simulink model "GPSRead"  (Simulink 6.6)
settings: Solver=FixedStepDiscrete  StartTime=0.0  StopTime=10.0  FixedStep=0.001  RelTol=1e-3
InitFcn:
  | initGPS
undefined symbols (not defined in the file or in its folder): gpsInit, gpsParse, gpsRead, gpsSeparate, u1, uartInit, y1
libraries: dsPICdrivers x13, simulink x1, xpclib x1
settings Model: Creator=ASL_Lab  LastModifiedBy=ASL_Lab  ProdHWDeviceType=16-bit Generic
settings OptimizationCC: InlineParams=on  OptimizeModelRefInitCode=on  LifeSpan=1
settings HardwareCC: ProdBitPerInt=16  ProdEndianess=LittleEndian  ProdWordSize=16  ProdHWDeviceType=16-bit Generic  TargetHWDeviceType=32-bit Generic
settings RTWCC: SystemTargetFile=dspic.tlc  TemplateMakefile=dspic_pic30_gcc.tmf  PostCodeGenCommand=dsPIC_Compile()  Description=Embedded Target for Microchip dsPIC (real-time)  GenerateReport=on  ProcessScript=dspic_make_rtw_hook  IncludeHyperlinkInReport=on  LaunchReport=on
settings RTWCC: CustomSource=|
  | clib\circBuffer.c
  | clib\gpsParse.c
  | clib\gpsSplit.c
  | clib\sbrk.c
  | clib\bufferedUART.c
settings CodeAppCC: IgnoreCustomStorageClasses=off
settings STFCustomTargetCC: TargetFcnLib=ansi_tfl_tmw.mat  GenFloatMathFcnCalls=ANSI_C  ModelReferenceCompliant=off  IncludeMdlTerminateFcn=off  CombineOutputUpdateFcns=on  SuppressErrorStatus=on  ERTCustomFileBanners=on  SupportContinuousTime=off  SupportNonInlinedSFcns=off  SystemTargetFile=dspic.tlc
settings ERTTargetCC: TargetFcnLib=ansi_tfl_tmw.mat  GenFloatMathFcnCalls=ANSI_C  ModelReferenceCompliant=off  IncludeMdlTerminateFcn=off  SuppressErrorStatus=on  ModelStepFunctionPrototypeControlCompliant=off  ExtModeMexFile=noextcomm  InlinedParameterPlacement=NonHierarchical  ERTSrcFileBannerTemplate=dsPIC_code_template.cgt  ERTHdrFileBannerTemplate=dsPIC_code_template.cgt  ERTDataSrcFileTemplate=dsPIC_code_template.cgt  ERTDataHdrFileTemplate=dsPIC_code_template.cgt  ERTCustomFileTemplate=dsPIC_main.tlc
settings CustomProperty: DataType=string  Value=C:\PROGRA~1\MATLAB\R2007a\rtw\bin\win32\gmake

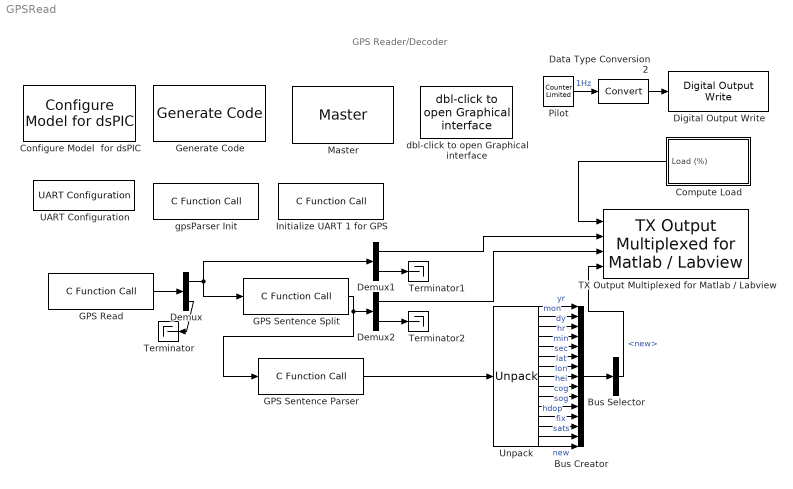
== system GPSRead ==
  note: GPS Reader/Decoder
  Bus Creator : BusCreator  Inputs=15
  Bus Selector : BusSelector  OutputSignals=new
  Compute Load : Subsystem  Orientation=left
  Configure Model  for dsPIC : dsPICdrivers/Simulink Configuration/Configure Model  for dsPIC
  Data Type Conversion2 : DataTypeConversion  OutDataTypeMode=boolean
  Demux : Demux  Outputs=[25 1]
  Demux1 : Demux  Outputs=[1 24]
  Demux2 : Demux  Outputs=[1 126]
  Digital Output Write : dsPICdrivers/Digital I//O/Digital Output Write  Tag=dsPIC_Digital_Output  Priority=5  PORT=G  Pin=[ 14]  Simultaneous=off  OrderingInOutPopup=None
  GPS Read : dsPICdrivers/OTHERS/C Function Call  Tag=dsPIC_dsPIC_CFunctionCall  fctName='gpsRead'  INPUT_SIZE=1  INPUT1=--  INPUT2=--  INPUT3=--  OUTPUT_SIZE=26  OUTPUT1=uint8  SampleTime=-1  InputType=[ ]  OutputType=[ 2 ]  FctDeclaration=extern void gpsRead(uint8_T* y1);  FctCall=gpsRead(*%y1);  OrderingInOutPopup=None
  GPS Sentence Parser : dsPICdrivers/OTHERS/C Function Call  Tag=dsPIC_dsPIC_CFunctionCall  fctName='gpsParse'  INPUT_SIZE=127  INPUT1=uint8  INPUT2=--  INPUT3=--  OUTPUT_SIZE=27  OUTPUT1=uint8  SampleTime=-1  InputType=[ 2 ]  OutputType=[ 2 ]  FctDeclaration=extern void gpsParse(uint8_T* u1,uint8_T* y1);  FctCall=gpsParse(*%u1, *%y1);  OrderingInOutPopup=None
  GPS Sentence Split : dsPICdrivers/OTHERS/C Function Call  Tag=dsPIC_dsPIC_CFunctionCall  fctName='gpsSeparate'  INPUT_SIZE=25  INPUT1=uint8  INPUT2=--  INPUT3=--  OUTPUT_SIZE=127  OUTPUT1=uint8  SampleTime=-1  InputType=[ 2 ]  OutputType=[ 2 ]  FctDeclaration=extern void gpsSeparate(uint8_T* u1,uint8_T* y1);  FctCall=gpsSeparate(*%u1, *%y1);  OrderingInOutPopup=None
  Generate Code : dsPICdrivers/Simulink Configuration/Generate Code
  Initialize UART 1 for GPS : dsPICdrivers/OTHERS/C Function Call  Tag=dsPIC_dsPIC_CFunctionCall  fctName='uartInit'  INPUT_SIZE=1  INPUT1=--  INPUT2=--  INPUT3=--  OUTPUT_SIZE=1  OUTPUT1=--  SampleTime=inf  InputType=[ ]  OutputType=[ ]  FctDeclaration=extern void uartInit();  FctCall=uartInit();  OrderingInOutPopup=None
  Master : dsPICdrivers/Master  Tag=dsPIC_MASTER  Priority=1  TimeStepType=Timer1  picType=33fJ256MC710  fcy=40000000  Quartz_33f=12e6  PLLActive_33f=on  fcyDesired_33f=40e6  tmr1="[1  39999  0]"  tmr1Info="Time Step : 0.001  ;   Error : 0%  PR1=39999"  tmr2345="[0  0  0  0  0  0  0  0]"  tmr2345cfg=[-1 -1 -1 -1 -1 -1 -1 -1]  IOautoConf=on  typePort="[ 0   0   0   0   0   0  10  10   0   0   0   0   0   0   0   0   0   0   0   0   0   0   0   0   0   0   0   0   0   0   0   0   0   0   0   0   0   0   0   0   0   0   0   0   0   0   0   0   0   0   0   0   0   0   0   0   0   0   0   0   0   0   0   0   0   0   0   0   0   0   0   0   0   0   0   0   0   0   0   0   0   0   0   0   4   5   0   0   0   0   0   0   0   0   0   0   0   0   0   0   0   0   0   0   0   0   0   0   0   0  10   0 ]"  TRIS="[ 65343  65535  65535  65535  65535  65535  49151 ]"  ADPCFG=12582912  MasterBusyPort=A7  MasterOverloadPort=A6  FOSC=Quartz (XT - HS)  TempProtection_33f=TEMP_ON  FPBOR=<empty>  PWRT=disable  MCLR=<empty>  PowerSave=off
  Pilot : simulink/Sources/Counter Limited  SystemSampleTime=-1  uplimit=1  tsamp=1.0
  TX Output Multiplexed for Matlab / Labview : dsPICdrivers/Serial PORT/TX Output Multiplexed for Matlab // Labview  Tag=dsPIC_TX_Multiplexed  Priority=5  UART=2  CleverSpreadingChk=on  CleverSpreading=1  CHANNEL="[0 1 2 3  ]"  CHANNELBLOCKED=[]  CHANNELBLOCKED_BITEWISE=0  Status=OK
  Terminator : Terminator
  Terminator1 : Terminator
  Terminator2 : Terminator
  UART Configuration : dsPICdrivers/Serial PORT/UART Configuration  Tag=dsPIC_config_UART  Priority=2  UART=2  proposed_BAUD=19200  ALT_TX_RX=off  InterruptTxWhen=When Transmit Buffer is empty  TXInterruptPri=6  TxBufferSize=64  TXEN=on  InterruptRxWhen=When Receive Buffer is full (contain 4 characters)  RXInterruptPri=5  RxBufferSize=64  BAUD=19200  UxBRG=129  Info="UxBRG = 129   ||  Real Baud : 19231   ||  % error : 0.16026  ||  max 1.9231 Bytes / Step"  RealBaud=0
  Unpack : xpclib/UDP/Unpack  dimensions={1,1,1,1,1,1,1,1,1,1,1,1,1,1,1}  datatypes={'uint8', 'uint8', 'uint8', 'uint8', 'uint8', 'uint8', 'single', 'single','single','uint16', 'uint16', 'uint16', 'uint8','uint8', 'uint8'}  byteAlign=1
  dbl-click to open Graphical interface : dsPICdrivers/Serial PORT/dbl-click to open Graphical interface  SystemSampleTime=-1  Nothing=0
  gpsParser Init : dsPICdrivers/OTHERS/C Function Call  Tag=dsPIC_dsPIC_CFunctionCall  fctName='gpsInit'  INPUT_SIZE=1  INPUT1=--  INPUT2=--  INPUT3=--  OUTPUT_SIZE=1  OUTPUT1=--  SampleTime=inf  InputType=[ ]  OutputType=[ ]  FctDeclaration=extern void gpsInit();  FctCall=gpsInit();  OrderingInOutPopup=None
  wires:
  Pilot/1 -> Data Type Conversion2/1  "1Hz"
  Data Type Conversion2/1 -> Digital Output Write/1
  Compute Load/1(Load (%)) -> TX Output Multiplexed for Matlab / Labview/1
  GPS Sentence Split/1 -> GPS Sentence Parser/1, Demux2/1
  GPS Sentence Parser/1 -> Unpack/1
  Unpack/1 -> Bus Creator/1  "yr"
  Unpack/2 -> Bus Creator/2  "mon"
  Unpack/3 -> Bus Creator/3  "dy"
  Unpack/4 -> Bus Creator/4  "hr"
  Unpack/5 -> Bus Creator/5  "min"
  Unpack/6 -> Bus Creator/6  "sec"
  Unpack/7 -> Bus Creator/7  "lat"
  Unpack/8 -> Bus Creator/8  "lon"
  Unpack/9 -> Bus Creator/9  "hei"
  Unpack/10 -> Bus Creator/10  "cog"
  Unpack/11 -> Bus Creator/11  "sog"
  Unpack/12 -> Bus Creator/12  "hdop"
  Unpack/13 -> Bus Creator/13  "fix"
  Unpack/14 -> Bus Creator/14  "sats"
  Bus Creator/1 -> Bus Selector/1
  GPS Read/1 -> Demux/1
  Demux/1 -> GPS Sentence Split/1, Demux1/1
  Demux/2 -> Terminator/1
  Demux1/2 -> Terminator1/1
  Demux1/1 -> TX Output Multiplexed for Matlab / Labview/2
  Unpack/15 -> Bus Creator/15  "new"
  Demux2/2 -> Terminator2/1
  Demux2/1 -> TX Output Multiplexed for Matlab / Labview/3
  Bus Selector/1 -> TX Output Multiplexed for Matlab / Labview/4  "<new>"

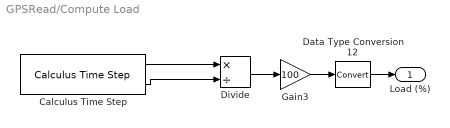
== system GPSRead/Compute Load ==
  Calculus Time Step : dsPICdrivers/OTHERS/Calculus Time Step  Tag=dsPIC_CalculusTimeStep  SampleTime=.005  PR1chk=on
  Data Type Conversion12 : DataTypeConversion  OutDataTypeMode=uint16
  Divide : Product  Inputs=*/  OutDataTypeMode=double  OutScaling=2^-10
  Gain3 : Gain  Gain=100
  Load (%) : Outport
  wires:
  Data Type Conversion12/1 -> Load (%)/1
  Gain3/1 -> Data Type Conversion12/1
  Divide/1 -> Gain3/1
  Calculus Time Step/2 -> Divide/2
  Calculus Time Step/1 -> Divide/1
